simulink model "SS_MIMO_U_MPCRobusto_Simulink"  (R2016b)
settings: Solver=VariableStepAuto  StartTime=0.0  StopTime=30  FixedStep=0.1  RelTol=1e-3
values from neighbouring files (symbols this model uses):
  Td = 0.1    [Initialization_MPC_SS.m]    (also in Script_identificacionW.m)
undefined symbols (not defined in the file or in its folder): nu, ny
settings Model: Creator=asierzubizarreta  LastModifiedBy=asierzubizarreta
settings DataIOCC: LimitDataPoints=on  SaveFormat=Array
settings OptimizationCC: BlockReduction=off  BooleanDataType=off  LifeSpan=inf
settings DebuggingCC: SaveWithParameterizedLinksMsg=none  UnderspecifiedInitializationDetection=Classic  MergeDetectMultiDrivingBlocksExec=none  SignalResolutionControl=TryResolveAllWithWarning  SFUnexpectedBacktrackingDiag=warning  SFNoUnconditionalDefaultTransitionDiag=warning  SFExecutionAtInitializationDiag=none
settings HardwareCC: ProdBitPerPointer=32  ProdBitPerSizeT=32  ProdBitPerPtrDiffT=32  ProdLargestAtomicFloat=None  ProdIntDivRoundTo=Undefined  ProdEndianess=Unspecified  ProdWordSize=32  ProdHWDeviceType=32-bit Generic  TargetUnknown=on
settings ModelReferenceCC: PropagateSignalLabelsOutOfModel=off
settings GRTTargetCC: TargetLangStandard=C89/C90 (ANSI)  GeneratePreprocessorConditionals=Disable all
settings ConfigComp: CovMetricSettings=dw  CovHtmlReporting=on  CovSaveCumulativeToWorkspaceVar=on  CovSaveSingleToWorkspaceVar=on  CovExternalEMLEnable=off  CovSFcnEnable=off

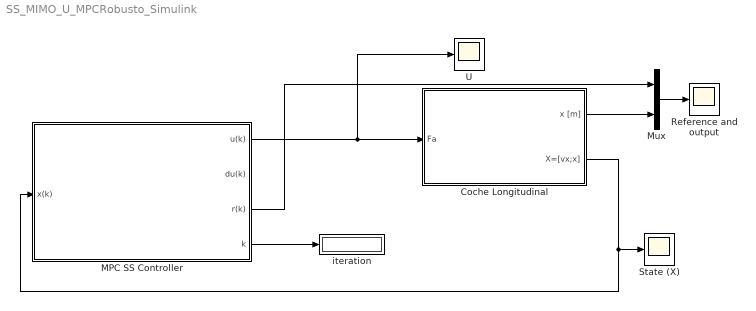
== system SS_MIMO_U_MPCRobusto_Simulink ==
  Coche Longitudinal : Subsystem  SystemSampleTime=Td  mask{m=1000, Br=500, Ka=50000, wlim1=1, wlim2=0.1, Td=0.1}
      mask prompts: m "Mass (m)"; Br "Friction (Br)"; Ka "Motor constant (Ka)"; wlim1 "Max Uncertainty (w_v)"; wlim2 "Max Uncertainty (w_x)"; Td "Discretization Time (Td)"
      mask init:
      | Ac=[-Br/m 0; 1 0];
      | Bc=[Ka/m;0];
      | Cc=eye(2);
      | 
      | %Dscretizaci?n
      | 
      | sc=ss(Ac,Bc,Cc,0);
      | 
      | %% Sistema discretizado:
      | 
      | sd=c2d(sc,Td);
      | A=sd.a;
      | B=sd.b;
      | C=sd.c;
  MPC SS Controller : Subsystem  InitFcn=|  TreatAsAtomicUnit=on  SystemSampleTime=Td
      | [parameters, Ref,Td]=Initialization_MPC_SS; 
      | [nx,nu]=size(parameters.B);
      | [ny,nx]=size(parameters.C);
      mask DialogControl DescGroupVar Prompt: MPC Controller
      mask Display:
      | fprintf('MPC SS Control\n\n\n');
      | 
      | 
      | port_label('output',1,'u(k)');
      | port_label('output',2,'du(k)');
      | port_label('output',3,'r(k)');
      | port_label('output',4,'k');
      | port_label('input',1,'x(k)');
  Mux : Mux  Inputs=2
  Reference and output : Scope
  State (X) : Scope
  U : Scope
  iteration : Display
  wires:
  Mux/1 -> Reference and output/1
  MPC SS Controller/1(u(k)) -> Coche Longitudinal/1(Fa), U/1
  MPC SS Controller/4(k) -> iteration/1
  MPC SS Controller/3(r(k)) -> Mux/1
  Coche Longitudinal/1(x [m]) -> Mux/2
  Coche Longitudinal/2(X=[vx;x]) -> MPC SS Controller/1(x(k)), State (X)/1

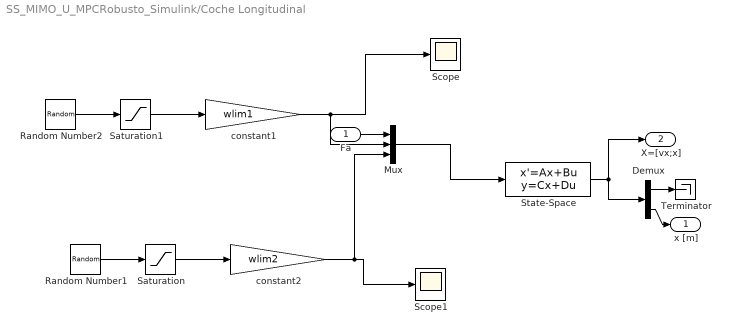
== system SS_MIMO_U_MPCRobusto_Simulink/Coche Longitudinal ==
  Fa : Inport
  Demux : Demux  Outputs=2
  Mux : Mux  Inputs=3
  Random Number1 : RandomNumber  Seed=1  SampleTime=0.1
  Random Number2 : RandomNumber  Seed=0.5  SampleTime=0.1
  Saturation : Saturate  UpperLimit=1  LowerLimit=-1
  Saturation1 : Saturate  UpperLimit=1  LowerLimit=-1
  Scope : Scope
  Scope1 : Scope
  State-Space : StateSpace  A=Ac  B=[Bc eye(2)]  C=eye(2)  D=zeros(2,3)  X0=0
  Terminator : Terminator
  constant1 : Gain  Gain=wlim1
  constant2 : Gain  Gain=wlim2
  x [m] : Outport
  X=[vx;x] : Outport  Port=2
  wires:
  Random Number1/1 -> Saturation/1
  constant1/1 -> Mux/2, Scope/1
  constant2/1 -> Mux/3, Scope1/1
  Demux/1 -> Terminator/1
  Demux/2 -> x [m]/1
  Random Number2/1 -> Saturation1/1
  Saturation1/1 -> constant1/1
  Saturation/1 -> constant2/1
  State-Space/1 -> X=[vx;x]/1, Demux/1
  Fa/1 -> Mux/1
  Mux/1 -> State-Space/1

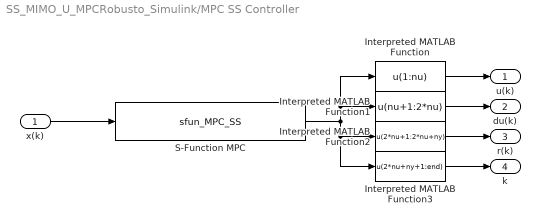
== system SS_MIMO_U_MPCRobusto_Simulink/MPC SS Controller ==
  x(k) : Inport
  Interpreted MATLAB Function : MATLABFcn  MATLABFcn=u(1:nu)
  Interpreted MATLAB Function1 : MATLABFcn  MATLABFcn=u(nu+1:2*nu)
  Interpreted MATLAB Function2 : MATLABFcn  MATLABFcn=u(2*nu+1:2*nu+ny)
  Interpreted MATLAB Function3 : MATLABFcn  MATLABFcn=u(2*nu+ny+1:end)
  S-Function MPC : S-Function  FunctionName=sfun_MPC_SS  SFunctionModules=s  SFunctionDeploymentMode=off  EnableBusSupport=off
  u(k) : Outport
  du(k) : Outport  Port=2
  r(k) : Outport  Port=3
  k : Outport  Port=4
  wires:
  Interpreted MATLAB Function/1 -> u(k)/1
  Interpreted MATLAB Function1/1 -> du(k)/1
  Interpreted MATLAB Function2/1 -> r(k)/1
  Interpreted MATLAB Function3/1 -> k/1
  x(k)/1 -> S-Function MPC/1
  S-Function MPC/1 -> Interpreted MATLAB Function1/1, Interpreted MATLAB Function/1, Interpreted MATLAB Function3/1, Interpreted MATLAB Function2/1
